simulink model "Quadcopter"  (R2024b)
settings: Solver=VariableStepAuto  StartTime=0.0  StopTime=50  RelTol=1e-3
undefined symbols (not defined in the file): g, I_xx, I_yy, I_zz, J_r, L, m, Omega_d, U_1, U_2, U_3, U_4
libraries: slpidlib x3
settings Model: Creator=sebas  LastModifiedBy=sebas

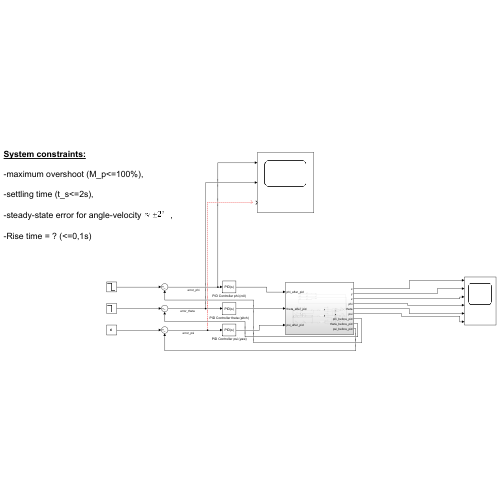
[thumbnail: Simulink's stored preview of the top-level diagram]
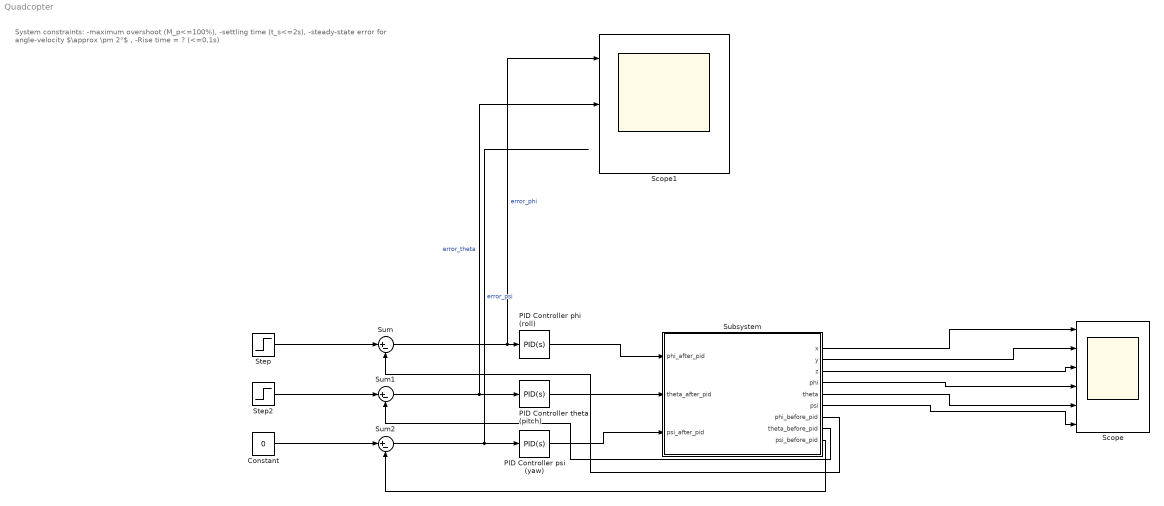
== system Quadcopter ==
  note: System constraints:
      |
      | -maximum overshoot (M_p<=100%),
      |
      | -settling time (t_s<=2s),
      |
      | -steady-state error for angle-velocity $\approx \pm 2°$ ,
      |
      | -Rise time = ? (<=0,1s)
  Constant : Constant  Value=0
  PID Controller phi (roll) : slpidlib/PID Controller  Controller=PID  Form=Parallel  TimeDomain=Continuous-time  UseExternalTs=off  SampleTime=-1  IntegratorMethod=Forward Euler  FilterMethod=Forward Euler  ControllerParametersSource=internal  P=1.32  I=0.05  UseKiTs=off  D=18.0  UseExternalDerivativeSource=off  N=100  UseFilter=on  TunerSelectOption=Transfer Function Based (PID Tuner App)  InitialConditionSource=internal  InitialConditionForIntegrator=0  InitialConditionForFilter=0  DifferentiatorICPrevScaledInput=0  ExternalReset=none  TrackingMode=off  Kt=1  LimitOutput=off  SatLimitsSource=internal  UpperSaturationLimit=inf  LowerSaturationLimit=-inf  LinearizeAsGain=on  AntiWindupMode=none  Kb=1  LimitIntegrator=off  UpperIntegratorSaturationLimit=inf  LowerIntegratorSaturationLimit=-inf  POutMin=[]  POutMax=[]  IOutMin=[]  IOutMax=[]  DOutMin=[]  DOutMax=[]  NOutMin=[]  NOutMax=[]  SumOutMin=[]  SumOutMax=[]  SaturationOutMin=[]  SaturationOutMax=[]  PParamMin=[]  PParamMax=[]  IParamMin=[]  IParamMax=[]  DParamMin=[]  DParamMax=[]  NParamMin=[]  NParamMax=[]  KbParamMin=[]  KbParamMax=[]  KtParamMin=[]  KtParamMax=[]  KbOutMin=[]  KbOutMax=[]  KtOutMin=[]  KtOutMax=[]  IntegratorOutMin=[]  IntegratorOutMax=[]  FilterOutMin=[]  FilterOutMax=[]  SumI1OutMin=[]  SumI1OutMax=[]  SumI2OutMin=[]  SumI2OutMax=[]  SumI3OutMin=[]  SumI3OutMax=[]  SumI4OutMin=[]  SumI4OutMax=[]  SumDOutMin=[]  SumDOutMax=[]  DifferentiatorOutMin=[]  DifferentiatorOutMax=[]  FilterDiffOutCoefMin=[]  FilterDiffOutCoefMax=[]  ReciprocalOutMin=[]  ReciprocalOutMax=[]  SumDenOutMin=[]  SumDenOutMax=[]  SumNumOutMin=[]  SumNumOutMax=[]  DivideOutMin=[]  DivideOutMax=[]  UdiffTsProdOutMin=[]  UdiffTsProdOutMax=[]  NTsProdOutMin=[]  NTsProdOutMax=[]  UintegralTsProdOutMin=[]  UintegralTsProdOutMax=[]  UngainTsProdOutMin=[]  UngainTsProdOutMax=[]  ClampingZeroOutDataTypeStr=Inherit: Inherit via back propagation  ClampingZeroOutMin=[]  ClampingZeroOutMax=[]  FilterDenConstantOutDataTypeStr=Inherit: Inherit via back propagation  FilterDenConstantOutMin=[]  FilterDenConstantOutMax=[]  PCopyOutDataTypeStr=Inherit: Inherit via back propagation  PCopyOutMin=[]  PCopyOutMax=[]  NCopyOutDataTypeStr=Inherit: Inherit via back propagation  NCopyOutMin=[]  NCopyOutMax=[]  IntegratorContinuousStateAttributes=''  IntegratorStateMustResolveToSignalObject=off  IntegratorRTWStateStorageClass=Auto  FilterContinuousStateAttributes=''  FilterStateMustResolveToSignalObject=off  FilterRTWStateStorageClass=Auto  ParallelPVariant=InternalParameters  IdealPVariant=Disabled  IVariant=InternalParameters  DVariant=InternalParameters  IntegratorVariant=Continuous  SatVariant=Disabled  AWVariant=Passthrough  PCopyVariant=Disabled  TRVariant=Disabled  FdbkBlocksVariant=Forward  IdealPFdbkVariant=Disabled  SatFdbkVariant=Disabled  DerivativeFilterVariant=ContFilter  NVariant=InternalParameters  NCopyVariant=Disabled  FilterICVariant=InternalICsFilter  IntegratorICVariant=InternalICs  ExternalResetVariant=Disabled  TRSumVariant=Passthrough  SumFdbkVariant=Disabled  SumVariant=Sum_PID  TsampFilterVariant=InternalTs  TsampNgainVariant=Passthrough  TsampIntegralVariant=Disabled_SignalSpec  ExternalSaturationOutDataTypeStr=Inherit: Same as second input  DerivativeSourceVariant=ErrorSignal  PreIntVariant=InternalPreInt
  PID Controller psi (yaw) : slpidlib/PID Controller  Controller=PID  Form=Parallel  TimeDomain=Continuous-time  UseExternalTs=off  SampleTime=-1  IntegratorMethod=Forward Euler  FilterMethod=Forward Euler  ControllerParametersSource=internal  P=4.11  I=0.03  UseKiTs=off  D=0  UseExternalDerivativeSource=off  N=100  UseFilter=on  TunerSelectOption=Transfer Function Based (PID Tuner App)  InitialConditionSource=internal  InitialConditionForIntegrator=0  InitialConditionForFilter=0  DifferentiatorICPrevScaledInput=0  ExternalReset=none  TrackingMode=off  Kt=1  LimitOutput=off  SatLimitsSource=internal  UpperSaturationLimit=inf  LowerSaturationLimit=-inf  LinearizeAsGain=on  AntiWindupMode=none  Kb=1  LimitIntegrator=off  UpperIntegratorSaturationLimit=inf  LowerIntegratorSaturationLimit=-inf  POutMin=[]  POutMax=[]  IOutMin=[]  IOutMax=[]  DOutMin=[]  DOutMax=[]  NOutMin=[]  NOutMax=[]  SumOutMin=[]  SumOutMax=[]  SaturationOutMin=[]  SaturationOutMax=[]  PParamMin=[]  PParamMax=[]  IParamMin=[]  IParamMax=[]  DParamMin=[]  DParamMax=[]  NParamMin=[]  NParamMax=[]  KbParamMin=[]  KbParamMax=[]  KtParamMin=[]  KtParamMax=[]  KbOutMin=[]  KbOutMax=[]  KtOutMin=[]  KtOutMax=[]  IntegratorOutMin=[]  IntegratorOutMax=[]  FilterOutMin=[]  FilterOutMax=[]  SumI1OutMin=[]  SumI1OutMax=[]  SumI2OutMin=[]  SumI2OutMax=[]  SumI3OutMin=[]  SumI3OutMax=[]  SumI4OutMin=[]  SumI4OutMax=[]  SumDOutMin=[]  SumDOutMax=[]  DifferentiatorOutMin=[]  DifferentiatorOutMax=[]  FilterDiffOutCoefMin=[]  FilterDiffOutCoefMax=[]  ReciprocalOutMin=[]  ReciprocalOutMax=[]  SumDenOutMin=[]  SumDenOutMax=[]  SumNumOutMin=[]  SumNumOutMax=[]  DivideOutMin=[]  DivideOutMax=[]  UdiffTsProdOutMin=[]  UdiffTsProdOutMax=[]  NTsProdOutMin=[]  NTsProdOutMax=[]  UintegralTsProdOutMin=[]  UintegralTsProdOutMax=[]  UngainTsProdOutMin=[]  UngainTsProdOutMax=[]  ClampingZeroOutDataTypeStr=Inherit: Inherit via back propagation  ClampingZeroOutMin=[]  ClampingZeroOutMax=[]  FilterDenConstantOutDataTypeStr=Inherit: Inherit via back propagation  FilterDenConstantOutMin=[]  FilterDenConstantOutMax=[]  PCopyOutDataTypeStr=Inherit: Inherit via back propagation  PCopyOutMin=[]  PCopyOutMax=[]  NCopyOutDataTypeStr=Inherit: Inherit via back propagation  NCopyOutMin=[]  NCopyOutMax=[]  IntegratorContinuousStateAttributes=''  IntegratorStateMustResolveToSignalObject=off  IntegratorRTWStateStorageClass=Auto  FilterContinuousStateAttributes=''  FilterStateMustResolveToSignalObject=off  FilterRTWStateStorageClass=Auto  ParallelPVariant=InternalParameters  IdealPVariant=Disabled  IVariant=InternalParameters  DVariant=InternalParameters  IntegratorVariant=Continuous  SatVariant=Disabled  AWVariant=Passthrough  PCopyVariant=Disabled  TRVariant=Disabled  FdbkBlocksVariant=Forward  IdealPFdbkVariant=Disabled  SatFdbkVariant=Disabled  DerivativeFilterVariant=ContFilter  NVariant=InternalParameters  NCopyVariant=Disabled  FilterICVariant=InternalICsFilter  IntegratorICVariant=InternalICs  ExternalResetVariant=Disabled  TRSumVariant=Passthrough  SumFdbkVariant=Disabled  SumVariant=Sum_PID  TsampFilterVariant=InternalTs  TsampNgainVariant=Passthrough  TsampIntegralVariant=Disabled_SignalSpec  ExternalSaturationOutDataTypeStr=Inherit: Same as second input  DerivativeSourceVariant=ErrorSignal  PreIntVariant=InternalPreInt
  PID Controller theta (pitch) : slpidlib/PID Controller  Controller=PID  Form=Parallel  TimeDomain=Continuous-time  UseExternalTs=off  SampleTime=-1  IntegratorMethod=Forward Euler  FilterMethod=Forward Euler  ControllerParametersSource=internal  P=1.30  I=0.05  UseKiTs=off  D=18.0  UseExternalDerivativeSource=off  N=100  UseFilter=on  TunerSelectOption=Transfer Function Based (PID Tuner App)  InitialConditionSource=internal  InitialConditionForIntegrator=0  InitialConditionForFilter=0  DifferentiatorICPrevScaledInput=0  ExternalReset=none  TrackingMode=off  Kt=1  LimitOutput=off  SatLimitsSource=internal  UpperSaturationLimit=inf  LowerSaturationLimit=-inf  LinearizeAsGain=on  AntiWindupMode=none  Kb=1  LimitIntegrator=off  UpperIntegratorSaturationLimit=inf  LowerIntegratorSaturationLimit=-inf  POutMin=[]  POutMax=[]  IOutMin=[]  IOutMax=[]  DOutMin=[]  DOutMax=[]  NOutMin=[]  NOutMax=[]  SumOutMin=[]  SumOutMax=[]  SaturationOutMin=[]  SaturationOutMax=[]  PParamMin=[]  PParamMax=[]  IParamMin=[]  IParamMax=[]  DParamMin=[]  DParamMax=[]  NParamMin=[]  NParamMax=[]  KbParamMin=[]  KbParamMax=[]  KtParamMin=[]  KtParamMax=[]  KbOutMin=[]  KbOutMax=[]  KtOutMin=[]  KtOutMax=[]  IntegratorOutMin=[]  IntegratorOutMax=[]  FilterOutMin=[]  FilterOutMax=[]  SumI1OutMin=[]  SumI1OutMax=[]  SumI2OutMin=[]  SumI2OutMax=[]  SumI3OutMin=[]  SumI3OutMax=[]  SumI4OutMin=[]  SumI4OutMax=[]  SumDOutMin=[]  SumDOutMax=[]  DifferentiatorOutMin=[]  DifferentiatorOutMax=[]  FilterDiffOutCoefMin=[]  FilterDiffOutCoefMax=[]  ReciprocalOutMin=[]  ReciprocalOutMax=[]  SumDenOutMin=[]  SumDenOutMax=[]  SumNumOutMin=[]  SumNumOutMax=[]  DivideOutMin=[]  DivideOutMax=[]  UdiffTsProdOutMin=[]  UdiffTsProdOutMax=[]  NTsProdOutMin=[]  NTsProdOutMax=[]  UintegralTsProdOutMin=[]  UintegralTsProdOutMax=[]  UngainTsProdOutMin=[]  UngainTsProdOutMax=[]  ClampingZeroOutDataTypeStr=Inherit: Inherit via back propagation  ClampingZeroOutMin=[]  ClampingZeroOutMax=[]  FilterDenConstantOutDataTypeStr=Inherit: Inherit via back propagation  FilterDenConstantOutMin=[]  FilterDenConstantOutMax=[]  PCopyOutDataTypeStr=Inherit: Inherit via back propagation  PCopyOutMin=[]  PCopyOutMax=[]  NCopyOutDataTypeStr=Inherit: Inherit via back propagation  NCopyOutMin=[]  NCopyOutMax=[]  IntegratorContinuousStateAttributes=''  IntegratorStateMustResolveToSignalObject=off  IntegratorRTWStateStorageClass=Auto  FilterContinuousStateAttributes=''  FilterStateMustResolveToSignalObject=off  FilterRTWStateStorageClass=Auto  ParallelPVariant=InternalParameters  IdealPVariant=Disabled  IVariant=InternalParameters  DVariant=InternalParameters  IntegratorVariant=Continuous  SatVariant=Disabled  AWVariant=Passthrough  PCopyVariant=Disabled  TRVariant=Disabled  FdbkBlocksVariant=Forward  IdealPFdbkVariant=Disabled  SatFdbkVariant=Disabled  DerivativeFilterVariant=ContFilter  NVariant=InternalParameters  NCopyVariant=Disabled  FilterICVariant=InternalICsFilter  IntegratorICVariant=InternalICs  ExternalResetVariant=Disabled  TRSumVariant=Passthrough  SumFdbkVariant=Disabled  SumVariant=Sum_PID  TsampFilterVariant=InternalTs  TsampNgainVariant=Passthrough  TsampIntegralVariant=Disabled_SignalSpec  ExternalSaturationOutDataTypeStr=Inherit: Same as second input  DerivativeSourceVariant=ErrorSignal  PreIntVariant=InternalPreInt
  Scope : Scope  NumInputPorts=6
  Scope1 : Scope  NumInputPorts=3
  Step : Step  Time=10  Before=30  After=0  SampleTime=0
  Step2 : Step  Time=10  Before=20  After=0  SampleTime=0
  Subsystem : Subsystem
  Sum : Sum  Inputs=|+-
  Sum1 : Sum  Inputs=|+-
  Sum2 : Sum  Inputs=|+-
  wires:
  Sum/1 -> Scope1/1, PID Controller phi (roll)/1  "error_phi"
  Sum1/1 -> Scope1/2, PID Controller theta (pitch)/1  "error_theta"
  Sum2/1 -> PID Controller psi (yaw)/1  "error_psi"
  PID Controller phi (roll)/1 -> Subsystem/1(phi_after_pid)
  PID Controller psi (yaw)/1 -> Subsystem/3(psi_after_pid)
  PID Controller theta (pitch)/1 -> Subsystem/2(theta_after_pid)
  Subsystem/1(x) -> Scope/1
  Subsystem/2(y) -> Scope/2
  Subsystem/3(z) -> Scope/3
  Subsystem/4(phi) -> Scope/4
  Subsystem/5(theta) -> Scope/5
  Subsystem/6(psi) -> Scope/6
  Step/1 -> Sum/1
  Step2/1 -> Sum1/1
  Constant/1 -> Sum2/1
  Subsystem/7(phi_before_pid) -> Sum/2
  Subsystem/8(theta_before_pid) -> Sum1/2
  Subsystem/9(psi_before_pid) -> Sum2/2

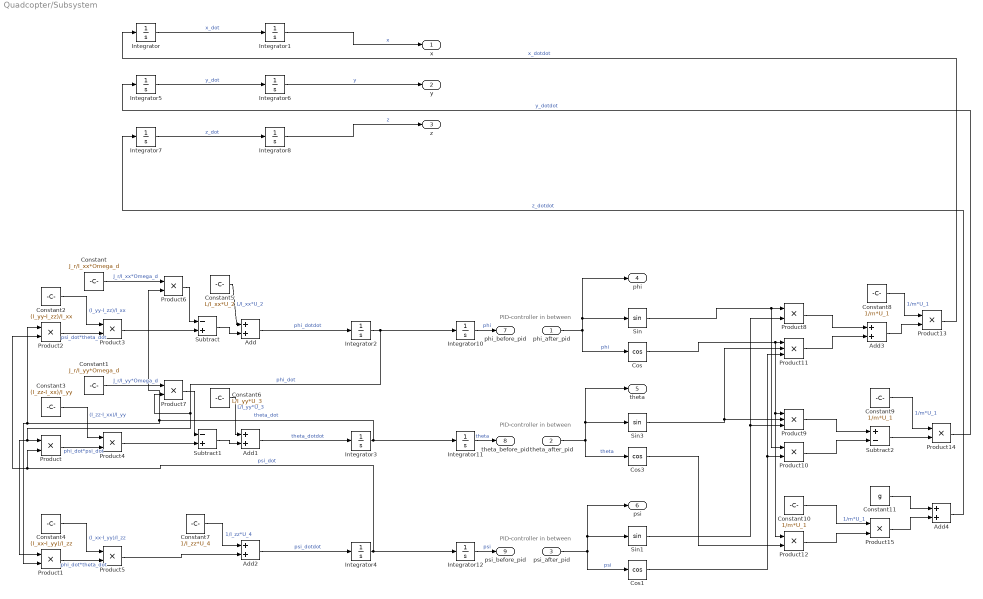
== system Quadcopter/Subsystem ==
  note: PID-controller in between
  note: PID-controller in between
  note: PID-controller in between
  phi_after_pid : Inport
  theta_after_pid : Inport  Port=2
  psi_after_pid : Inport  Port=3
  Add{,1..4} (5 alike) : Sum
  Constant : Constant  Value=J_r/I_xx*Omega_d
  Constant1 : Constant  Value=J_r/I_yy*Omega_d
  Constant10 : Constant  Value=1/m*U_1
  Constant11 : Constant  Value=g
  Constant2 : Constant  Value=(I_yy-I_zz)/I_xx
  Constant3 : Constant  Value=(I_zz-I_xx)/I_yy
  Constant4 : Constant  Value=(I_xx-I_yy)/I_zz
  Constant5 : Constant  Value=L/I_xx*U_2
  Constant6 : Constant  Value=L/I_yy*U_3
  Constant7 : Constant  Value=1/I_zz*U_4
  Constant8 : Constant  Value=1/m*U_1
  Constant9 : Constant  Value=1/m*U_1
  Cos : Trigonometry  Operator=cos
  Cos1 : Trigonometry  Operator=cos
  Cos3 : Trigonometry  Operator=cos
  Integrator{,1..8,12} (10 alike) : Integrator
  Integrator10 : Integrator  InitialCondition=30
  Integrator11 : Integrator  InitialCondition=20
  Product{,1..8,10,12..15} (14 alike) : Product
  Product11 : Product  Inputs=3
  Product9 : Product  Inputs=3
  Sin : Trigonometry
  Sin1 : Trigonometry
  Sin3 : Trigonometry
  Subtract : Sum  Inputs=-+
  Subtract1 : Sum  Inputs=-+
  Subtract2 : Sum  Inputs=+-
  x : Outport
  y : Outport  Port=2
  z : Outport  Port=3
  phi : Outport  Port=4
  theta : Outport  Port=5
  psi : Outport  Port=6
  phi_before_pid : Outport  Port=7
  theta_before_pid : Outport  Port=8
  psi_before_pid : Outport  Port=9
  wires:
  Constant3/1 -> Product4/1  "(I_zz-I_xx)/I_yy"
  Integrator3/1 -> Product6/2, Product1/2, Product2/1, Integrator11/1  "theta_dot"
  Constant11/1 -> Add4/1
  Integrator6/1 -> y/1  "y"
  Integrator4/1 -> Product/2, Product2/2, Integrator12/1  "psi_dot"
  Integrator2/1 -> Product7/2, Product1/1, Product/1, Integrator10/1  "phi_dot"
  Constant10/1 -> Product15/1  "1/m*U_1"
  Integrator7/1 -> Integrator8/1  "z_dot"
  Product6/1 -> Subtract/1
  Add4/1 -> Integrator7/1  "z_dotdot"
  Cos/1 -> Product9/1, Product12/1, Product11/1
  Cos1/1 -> Product10/2, Product11/3
  Constant5/1 -> Add/1  "L/I_xx*U_2"
  Constant7/1 -> Add2/1  "1/I_zz*U_4"
  Constant4/1 -> Product5/1  "(I_xx-I_yy)/I_zz"
  Product3/1 -> Subtract/2
  Subtract/1 -> Add/2
  Integrator8/1 -> z/1  "z"
  Sin/1 -> Product8/1, Product10/1
  Add1/1 -> Integrator3/1  "theta_dotdot"
  Add/1 -> Integrator2/1  "phi_dotdot"
  Product/1 -> Product4/2  "phi_dot*psi_dot"
  Product2/1 -> Product3/2  "psi_dot*theta_dot"
  Constant2/1 -> Product3/1  "(I_yy-I_zz)/I_xx"
  Subtract1/1 -> Add1/2
  Product8/1 -> Add3/1
  Product1/1 -> Product5/2  "phi_dot*theta_dot"
  Sin3/1 -> Product9/2, Product11/2
  Sin1/1 -> Product9/3, Product8/2
  Product15/1 -> Add4/2
  Add2/1 -> Integrator4/1  "psi_dotdot"
  Product4/1 -> Subtract1/2
  Cos3/1 -> Product12/2
  Product14/1 -> Integrator5/1  "y_dotdot"
  psi_after_pid/1 -> Sin1/1, psi/1, Cos1/1  "psi"
  Constant9/1 -> Product14/1  "1/m*U_1"
  Constant8/1 -> Product13/1  "1/m*U_1"
  Product12/1 -> Product15/2
  Product7/1 -> Subtract1/1
  Constant1/1 -> Product7/1  "J_r/I_yy*Omega_d"
  Integrator5/1 -> Integrator6/1  "y_dot"
  Product10/1 -> Subtract2/2
  Constant/1 -> Product6/1  "J_r/I_xx*Omega_d"
  Add3/1 -> Product13/2
  Product5/1 -> Add2/2
  Subtract2/1 -> Product14/2
  Product9/1 -> Subtract2/1
  Constant6/1 -> Add1/1  "L/I_yy*U_3"
  phi_after_pid/1 -> Sin/1, phi/1, Cos/1  "phi"
  Integrator1/1 -> x/1  "x"
  Product13/1 -> Integrator/1  "x_dotdot"
  theta_after_pid/1 -> Sin3/1, theta/1, Cos3/1  "theta"
  Integrator/1 -> Integrator1/1  "x_dot"
  Product11/1 -> Add3/2
  Integrator10/1 -> phi_before_pid/1  "phi"
  Integrator11/1 -> theta_before_pid/1  "theta"
  Integrator12/1 -> psi_before_pid/1  "psi"
